simulink model "PIDDiscrete"  (R2023a)
settings: Solver=FixedStepAuto  StartTime=0.0  StopTime=10.0  FixedStep=1e-3  MaxStep=1e-3  RelTol=1e-3
libraries: simulink x1
settings Model: Creator=Egypt_Laptop  LastModifiedBy=Egypt_Laptop

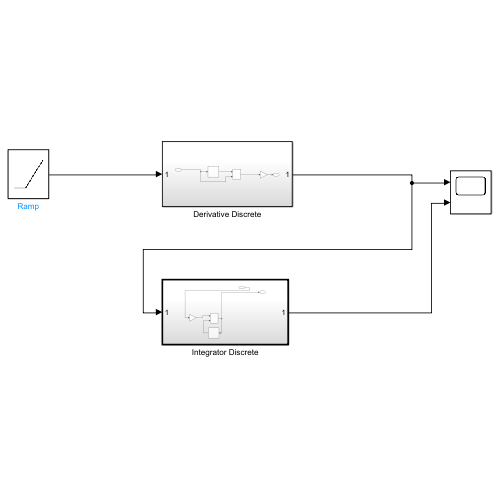
[thumbnail: Simulink's stored preview of the top-level diagram]
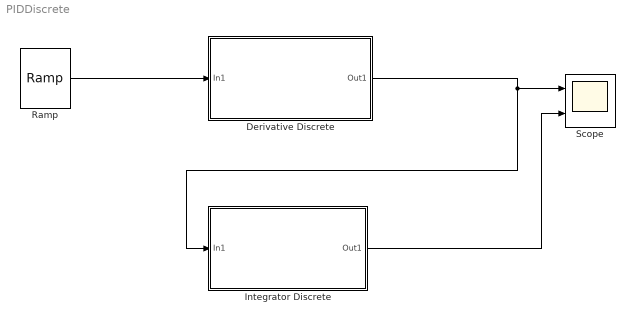
== system PIDDiscrete ==
  Derivative Discrete : Subsystem
  Integrator Discrete : Subsystem  TreatAsAtomicUnit=on
  Ramp : simulink/Sources/Ramp  slope=1  start=0  InitialOutput=0
  Scope : Scope  NumInputPorts=2
  wires:
  Derivative Discrete/1(Out1) -> Integrator Discrete/1(In1), Scope/1
  Ramp/1 -> Derivative Discrete/1(In1)
  Integrator Discrete/1(Out1) -> Scope/2

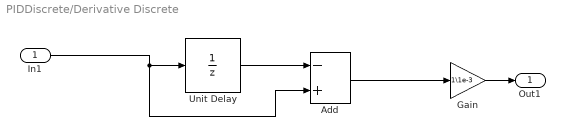
== system PIDDiscrete/Derivative Discrete ==
  In1 : Inport
  Add : Sum  Inputs=-+
  Gain : Gain  Gain=1\1e-3
  Unit Delay : UnitDelay  SampleTime=-1  HasFrameUpgradeWarning=on
  Out1 : Outport
  wires:
  In1/1 -> Add/2, Unit Delay/1
  Gain/1 -> Out1/1
  Add/1 -> Gain/1
  Unit Delay/1 -> Add/1

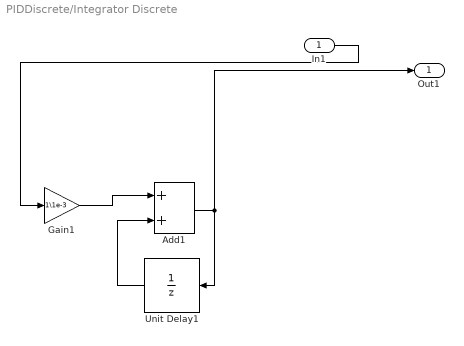
== system PIDDiscrete/Integrator Discrete ==
  In1 : Inport
  Add1 : Sum
  Gain1 : Gain  Gain=1\1e-3
  Unit Delay1 : UnitDelay  SampleTime=-1  HasFrameUpgradeWarning=on
  Out1 : Outport
  wires:
  Add1/1 -> Unit Delay1/1, Out1/1
  Unit Delay1/1 -> Add1/2
  Gain1/1 -> Add1/1
  In1/1 -> Gain1/1
